simulink model "EPT"  (R2019b)
settings: Solver=FixedStepDiscrete  StartTime=0.0  StopTime=5  FixedStep=0.005  RelTol=1e-3  EnableMultiTasking=on
PreLoadFcn:
  | try, model_open; catch, disp('Error occurred while executing model pre-load callback: model_open.m'); disp('Please assure that the MATLAB working directory is set to the model directory before opening.'); end
InitFcn:
  | try, model_open; catch, end
undefined symbols (not defined in the file or in its folder): Bridge, GCM, H, ln, raptor_get_param_eval, raptor_get_safe_string, raptor_xcp_function
libraries: Raptor_lib x2810, simulink x374, hdlsllib x19
(part 27 of 45)

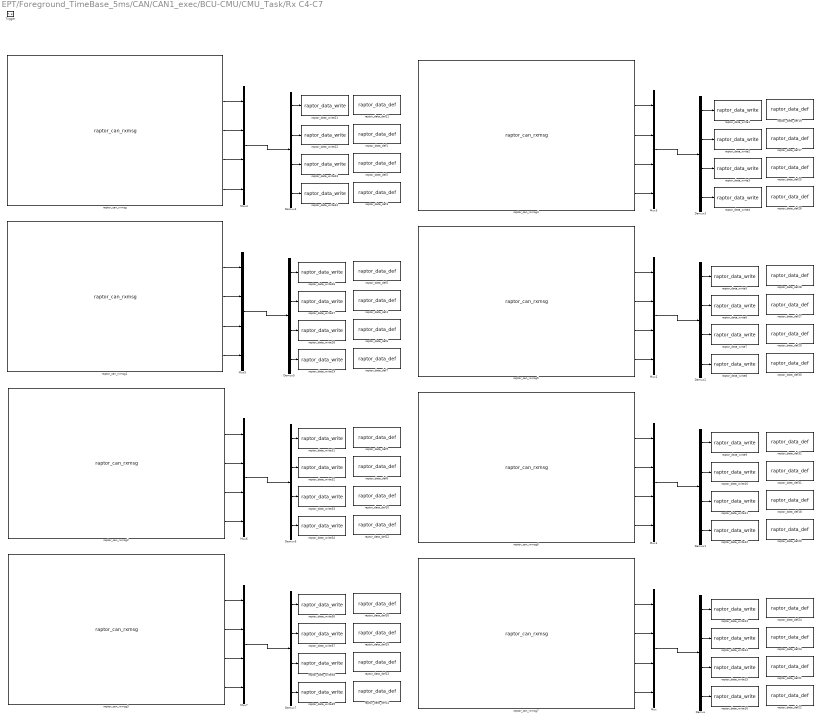
== system EPT/Foreground_TimeBase_5ms/CAN/CAN1_exec/BCU-CMU/CMU_Task/Rx C4-C7 ==
  Trigger : TriggerPort  VariantControl=Variant  PortDimensions=1
  Demux{,1..7} (8 alike) : Demux
  Mux{,1..7} (8 alike) : Mux
  raptor_can_rxmsg : Raptor_lib/CAN/raptor_can_rxmsg  canDefinition=struct('dbcFile', 'CMU1.dbc','message', 'Cell_Temp1','comment', '','signals', {{'Temp1','Temp2','Temp3','Temp4'}},'enabled', [ 1 1 1 1;],'canBus', '''CAN1''','messageID', [ 33604769;],'idMask', [ 536870911;],'payloadMask', [],'payloadValue', [],'period', [ 0;],'mailbox', '''''','queueSize', [ 1;],'label', [ 0;],'ver', [ 2;],'showID', [ 0;],'showRaw', [ 0;],'fill', [ 0;],'editID', [ 0;],'signalOrder', [ 2;])  canBus='CAN1'  mailbox=''  payloadMask=[]  payloadValue=[]  idMask=hex2dec('1FFFFFFF')  queueSize=1  showID=0  label=0  fill=0  id=33604769  showRaw=0  showAge=1  signalOrder=2  signalInfo={{struct('Name', 'Temp1','Startbit', [ 0;],'SignalSize', [ 16;],'ByteOrder', 'BigEndian','ValueType', 'UNSIGNED','Class', 'uint16','Signed', [ 0;],'Factor', [ 0.1;],'Offset', [ -40;],'Min', [ 0;],'Max', [ 0;],'Units', '','Comment', '','StartBit', [ 8;]),struct('Name', 'Temp2','Startbit', [ 0;],'SignalSize', [ 16;],'ByteOrder', 'BigEndian','ValueType', 'UNSIGNED','Class', 'uint16','Signed', [ 0;],'Factor', [ 0.1;],'Offset', [ -40;],'Min', [ 0;],'Max', [ 0;],'Units', '','Comment', '','StartBit', [ 24;]),struct('Name', 'Temp3','Startbit', [ 0;],'SignalSize', [ 16;],'ByteOrder', 'BigEndian','ValueType', 'UNSIGNED','Class', 'uint16','Signed', [ 0;],'Factor', [ 0.1;],'Offset', [ -40;],'Min', [ 0;],'Max', [ 0;],'Units', '','Comment', '','StartBit', [ 40;]),struct('Name', 'Temp4','Startbit', [ 0;],'SignalSize', [ 16;],'ByteOrder', 'BigEndian','ValueType', 'UNSIGNED','Class', 'uint16','Signed', [ 0;],'Factor', [ 0.1;],'Offset', [ -40;],'Min', [ 0;],'Max', [ 0;],'Units', '','Comment', '','StartBit', [ 56;])}}
      settings: SourceProductName=Raptor
  raptor_can_rxmsg1 : Raptor_lib/CAN/raptor_can_rxmsg  canDefinition=struct('dbcFile', 'CMU1.dbc','message', 'Cell_Temp2','comment', '','signals', {{'Temp5','Temp6','Temp7','Temp8'}},'enabled', [ 1 1 1 1;],'canBus', '''CAN1''','messageID', [ 33605025;],'idMask', [ 536870911;],'payloadMask', [],'payloadValue', [],'period', [ 0;],'mailbox', '''''','queueSize', [ 1;],'label', [ 0;],'ver', [ 2;],'showID', [ 0;],'showRaw', [ 0;],'fill', [ 0;],'editID', [ 0;],'signalOrder', [ 2;])  canBus='CAN1'  mailbox=''  payloadMask=[]  payloadValue=[]  idMask=hex2dec('1FFFFFFF')  queueSize=1  showID=0  label=0  fill=0  id=33605025  showRaw=0  showAge=1  signalOrder=2  signalInfo={{struct('Name', 'Temp5','Startbit', [ 0;],'SignalSize', [ 16;],'ByteOrder', 'BigEndian','ValueType', 'UNSIGNED','Class', 'uint16','Signed', [ 0;],'Factor', [ 0.1;],'Offset', [ -40;],'Min', [ 0;],'Max', [ 0;],'Units', '','Comment', '','StartBit', [ 8;]),struct('Name', 'Temp6','Startbit', [ 0;],'SignalSize', [ 16;],'ByteOrder', 'BigEndian','ValueType', 'UNSIGNED','Class', 'uint16','Signed', [ 0;],'Factor', [ 0.1;],'Offset', [ -40;],'Min', [ 0;],'Max', [ 0;],'Units', '','Comment', '','StartBit', [ 24;]),struct('Name', 'Temp7','Startbit', [ 0;],'SignalSize', [ 16;],'ByteOrder', 'BigEndian','ValueType', 'UNSIGNED','Class', 'uint16','Signed', [ 0;],'Factor', [ 0.1;],'Offset', [ -40;],'Min', [ 0;],'Max', [ 0;],'Units', '','Comment', '','StartBit', [ 40;]),struct('Name', 'Temp8','Startbit', [ 0;],'SignalSize', [ 16;],'ByteOrder', 'BigEndian','ValueType', 'UNSIGNED','Class', 'uint16','Signed', [ 0;],'Factor', [ 0.1;],'Offset', [ -40;],'Min', [ 0;],'Max', [ 0;],'Units', '','Comment', '','StartBit', [ 56;])}}
      settings: SourceProductName=Raptor
  raptor_can_rxmsg2 : Raptor_lib/CAN/raptor_can_rxmsg  canDefinition=struct('dbcFile', 'CMU1.dbc','message', 'Cell_Temp3','comment', '','signals', {{'Temp9','Temp10','Temp11','Temp12'}},'enabled', [ 1 1 1 1;],'canBus', '''CAN1''','messageID', [ 33605281;],'idMask', [ 536870911;],'payloadMask', [],'payloadValue', [],'period', [ 0;],'mailbox', '''''','queueSize', [ 1;],'label', [ 0;],'ver', [ 2;],'showID', [ 0;],'showRaw', [ 0;],'fill', [ 0;],'editID', [ 0;],'signalOrder', [ 2;])  canBus='CAN1'  mailbox=''  payloadMask=[]  payloadValue=[]  idMask=hex2dec('1FFFFFFF')  queueSize=1  showID=0  label=0  fill=0  id=33605281  showRaw=0  showAge=1  signalOrder=2  signalInfo={{struct('Name', 'Temp9','Startbit', [ 0;],'SignalSize', [ 16;],'ByteOrder', 'BigEndian','ValueType', 'UNSIGNED','Class', 'uint16','Signed', [ 0;],'Factor', [ 0.1;],'Offset', [ -40;],'Min', [ 0;],'Max', [ 0;],'Units', '','Comment', '','StartBit', [ 8;]),struct('Name', 'Temp10','Startbit', [ 0;],'SignalSize', [ 16;],'ByteOrder', 'BigEndian','ValueType', 'UNSIGNED','Class', 'uint16','Signed', [ 0;],'Factor', [ 0.1;],'Offset', [ -40;],'Min', [ 0;],'Max', [ 0;],'Units', '','Comment', '','StartBit', [ 24;]),struct('Name', 'Temp11','Startbit', [ 0;],'SignalSize', [ 16;],'ByteOrder', 'BigEndian','ValueType', 'UNSIGNED','Class', 'uint16','Signed', [ 0;],'Factor', [ 0.1;],'Offset', [ -40;],'Min', [ 0;],'Max', [ 0;],'Units', '','Comment', '','StartBit', [ 40;]),struct('Name', 'Temp12','Startbit', [ 0;],'SignalSize', [ 16;],'ByteOrder', 'BigEndian','ValueType', 'UNSIGNED','Class', 'uint16','Signed', [ 0;],'Factor', [ 0.1;],'Offset', [ -40;],'Min', [ 0;],'Max', [ 0;],'Units', '','Comment', '','StartBit', [ 56;])}}
      settings: SourceProductName=Raptor
  raptor_can_rxmsg3 : Raptor_lib/CAN/raptor_can_rxmsg  canDefinition=struct('dbcFile', 'CMU1.dbc','message', 'Cell_Temp4','comment', '','signals', {{'Temp13','Temp14','Temp15','Temp16'}},'enabled', [ 1 1 1 1;],'canBus', '''CAN1''','messageID', [ 33605537;],'idMask', [ 536870911;],'payloadMask', [],'payloadValue', [],'period', [ 0;],'mailbox', '''''','queueSize', [ 1;],'label', [ 0;],'ver', [ 2;],'showID', [ 0;],'showRaw', [ 0;],'fill', [ 0;],'editID', [ 0;],'signalOrder', [ 1;])  canBus='CAN1'  mailbox=''  payloadMask=[]  payloadValue=[]  idMask=hex2dec('1FFFFFFF')  queueSize=1  showID=0  label=0  fill=0  id=33605537  showRaw=0  showAge=1  signalOrder=1  signalInfo={{struct('Name', 'Temp13','Startbit', [ 0;],'SignalSize', [ 16;],'ByteOrder', 'BigEndian','ValueType', 'UNSIGNED','Class', 'uint16','Signed', [ 0;],'Factor', [ 0.1;],'Offset', [ -40;],'Min', [ 0;],'Max', [ 0;],'Units', '','Comment', '','StartBit', [ 8;]),struct('Name', 'Temp14','Startbit', [ 0;],'SignalSize', [ 16;],'ByteOrder', 'BigEndian','ValueType', 'UNSIGNED','Class', 'uint16','Signed', [ 0;],'Factor', [ 0.1;],'Offset', [ -40;],'Min', [ 0;],'Max', [ 0;],'Units', '','Comment', '','StartBit', [ 24;]),struct('Name', 'Temp15','Startbit', [ 0;],'SignalSize', [ 16;],'ByteOrder', 'BigEndian','ValueType', 'UNSIGNED','Class', 'uint16','Signed', [ 0;],'Factor', [ 0.1;],'Offset', [ -40;],'Min', [ 0;],'Max', [ 0;],'Units', '','Comment', '','StartBit', [ 40;]),struct('Name', 'Temp16','Startbit', [ 0;],'SignalSize', [ 16;],'ByteOrder', 'BigEndian','ValueType', 'UNSIGNED','Class', 'uint16','Signed', [ 0;],'Factor', [ 0.1;],'Offset', [ -40;],'Min', [ 0;],'Max', [ 0;],'Units', '','Comment', '','StartBit', [ 56;])}}
      settings: SourceProductName=Raptor
  raptor_can_rxmsg4 : Raptor_lib/CAN/raptor_can_rxmsg  canDefinition=struct('dbcFile', 'CMU2.dbc','message', 'Cell_Temp1','comment', '','signals', {{'Temp1','Temp2','Temp3','Temp4'}},'enabled', [ 1 1 1 1;],'canBus', '''CAN1''','messageID', [ 33604770;],'idMask', [ 536870911;],'payloadMask', [],'payloadValue', [],'period', [ 0;],'mailbox', '''''','queueSize', [ 1;],'label', [ 0;],'ver', [ 2;],'showID', [ 0;],'showRaw', [ 0;],'fill', [ 0;],'editID', [ 0;],'signalOrder', [ 2;])  canBus='CAN1'  mailbox=''  payloadMask=[]  payloadValue=[]  idMask=hex2dec('1FFFFFFF')  queueSize=1  showID=0  label=0  fill=0  id=33604770  showRaw=0  showAge=1  signalOrder=2  signalInfo={{struct('Name', 'Temp1','Startbit', [ 0;],'SignalSize', [ 16;],'ByteOrder', 'BigEndian','ValueType', 'UNSIGNED','Class', 'uint16','Signed', [ 0;],'Factor', [ 0.1;],'Offset', [ -40;],'Min', [ 0;],'Max', [ 0;],'Units', '','Comment', '','StartBit', [ 8;]),struct('Name', 'Temp2','Startbit', [ 0;],'SignalSize', [ 16;],'ByteOrder', 'BigEndian','ValueType', 'UNSIGNED','Class', 'uint16','Signed', [ 0;],'Factor', [ 0.1;],'Offset', [ -40;],'Min', [ 0;],'Max', [ 0;],'Units', '','Comment', '','StartBit', [ 24;]),struct('Name', 'Temp3','Startbit', [ 0;],'SignalSize', [ 16;],'ByteOrder', 'BigEndian','ValueType', 'UNSIGNED','Class', 'uint16','Signed', [ 0;],'Factor', [ 0.1;],'Offset', [ -40;],'Min', [ 0;],'Max', [ 0;],'Units', '','Comment', '','StartBit', [ 40;]),struct('Name', 'Temp4','Startbit', [ 0;],'SignalSize', [ 16;],'ByteOrder', 'BigEndian','ValueType', 'UNSIGNED','Class', 'uint16','Signed', [ 0;],'Factor', [ 0.1;],'Offset', [ -40;],'Min', [ 0;],'Max', [ 0;],'Units', '','Comment', '','StartBit', [ 56;])}}
      settings: SourceProductName=Raptor
  raptor_can_rxmsg5 : Raptor_lib/CAN/raptor_can_rxmsg  canDefinition=struct('dbcFile', 'CMU2.dbc','message', 'Cell_Temp2','comment', '','signals', {{'Temp5','Temp6','Temp7','Temp8'}},'enabled', [ 1 1 1 1;],'canBus', '''CAN1''','messageID', [ 33605026;],'idMask', [ 536870911;],'payloadMask', [],'payloadValue', [],'period', [ 0;],'mailbox', '''''','queueSize', [ 1;],'label', [ 0;],'ver', [ 2;],'showID', [ 0;],'showRaw', [ 0;],'fill', [ 0;],'editID', [ 0;],'signalOrder', [ 2;])  canBus='CAN1'  mailbox=''  payloadMask=[]  payloadValue=[]  idMask=hex2dec('1FFFFFFF')  queueSize=1  showID=0  label=0  fill=0  id=33605026  showRaw=0  showAge=1  signalOrder=2  signalInfo={{struct('Name', 'Temp5','Startbit', [ 0;],'SignalSize', [ 16;],'ByteOrder', 'BigEndian','ValueType', 'UNSIGNED','Class', 'uint16','Signed', [ 0;],'Factor', [ 0.1;],'Offset', [ -40;],'Min', [ 0;],'Max', [ 0;],'Units', '','Comment', '','StartBit', [ 8;]),struct('Name', 'Temp6','Startbit', [ 0;],'SignalSize', [ 16;],'ByteOrder', 'BigEndian','ValueType', 'UNSIGNED','Class', 'uint16','Signed', [ 0;],'Factor', [ 0.1;],'Offset', [ -40;],'Min', [ 0;],'Max', [ 0;],'Units', '','Comment', '','StartBit', [ 24;]),struct('Name', 'Temp7','Startbit', [ 0;],'SignalSize', [ 16;],'ByteOrder', 'BigEndian','ValueType', 'UNSIGNED','Class', 'uint16','Signed', [ 0;],'Factor', [ 0.1;],'Offset', [ -40;],'Min', [ 0;],'Max', [ 0;],'Units', '','Comment', '','StartBit', [ 40;]),struct('Name', 'Temp8','Startbit', [ 0;],'SignalSize', [ 16;],'ByteOrder', 'BigEndian','ValueType', 'UNSIGNED','Class', 'uint16','Signed', [ 0;],'Factor', [ 0.1;],'Offset', [ -40;],'Min', [ 0;],'Max', [ 0;],'Units', '','Comment', '','StartBit', [ 56;])}}
      settings: SourceProductName=Raptor
  raptor_can_rxmsg6 : Raptor_lib/CAN/raptor_can_rxmsg  canDefinition=struct('dbcFile', 'CMU2.dbc','message', 'Cell_Temp3','comment', '','signals', {{'Temp9','Temp10','Temp11','Temp12'}},'enabled', [ 1 1 1 1;],'canBus', '''CAN1''','messageID', [ 33605282;],'idMask', [ 536870911;],'payloadMask', [],'payloadValue', [],'period', [ 0;],'mailbox', '''''','queueSize', [ 1;],'label', [ 0;],'ver', [ 2;],'showID', [ 0;],'showRaw', [ 0;],'fill', [ 0;],'editID', [ 0;],'signalOrder', [ 2;])  canBus='CAN1'  mailbox=''  payloadMask=[]  payloadValue=[]  idMask=hex2dec('1FFFFFFF')  queueSize=1  showID=0  label=0  fill=0  id=33605282  showRaw=0  showAge=1  signalOrder=2  signalInfo={{struct('Name', 'Temp9','Startbit', [ 0;],'SignalSize', [ 16;],'ByteOrder', 'BigEndian','ValueType', 'UNSIGNED','Class', 'uint16','Signed', [ 0;],'Factor', [ 0.1;],'Offset', [ -40;],'Min', [ 0;],'Max', [ 0;],'Units', '','Comment', '','StartBit', [ 8;]),struct('Name', 'Temp10','Startbit', [ 0;],'SignalSize', [ 16;],'ByteOrder', 'BigEndian','ValueType', 'UNSIGNED','Class', 'uint16','Signed', [ 0;],'Factor', [ 0.1;],'Offset', [ -40;],'Min', [ 0;],'Max', [ 0;],'Units', '','Comment', '','StartBit', [ 24;]),struct('Name', 'Temp11','Startbit', [ 0;],'SignalSize', [ 16;],'ByteOrder', 'BigEndian','ValueType', 'UNSIGNED','Class', 'uint16','Signed', [ 0;],'Factor', [ 0.1;],'Offset', [ -40;],'Min', [ 0;],'Max', [ 0;],'Units', '','Comment', '','StartBit', [ 40;]),struct('Name', 'Temp12','Startbit', [ 0;],'SignalSize', [ 16;],'ByteOrder', 'BigEndian','ValueType', 'UNSIGNED','Class', 'uint16','Signed', [ 0;],'Factor', [ 0.1;],'Offset', [ -40;],'Min', [ 0;],'Max', [ 0;],'Units', '','Comment', '','StartBit', [ 56;])}}
      settings: SourceProductName=Raptor
  raptor_can_rxmsg7 : Raptor_lib/CAN/raptor_can_rxmsg  canDefinition=struct('dbcFile', 'CMU2.dbc','message', 'Cell_Temp4','comment', '','signals', {{'Temp13','Temp14','Temp15','Temp16'}},'enabled', [ 1 1 1 1;],'canBus', '''CAN1''','messageID', [ 33605538;],'idMask', [ 536870911;],'payloadMask', [],'payloadValue', [],'period', [ 0;],'mailbox', '''''','queueSize', [ 1;],'label', [ 0;],'ver', [ 2;],'showID', [ 0;],'showRaw', [ 0;],'fill', [ 0;],'editID', [ 0;],'signalOrder', [ 2;])  canBus='CAN1'  mailbox=''  payloadMask=[]  payloadValue=[]  idMask=hex2dec('1FFFFFFF')  queueSize=1  showID=0  label=0  fill=0  id=33605538  showRaw=0  showAge=1  signalOrder=2  signalInfo={{struct('Name', 'Temp13','Startbit', [ 0;],'SignalSize', [ 16;],'ByteOrder', 'BigEndian','ValueType', 'UNSIGNED','Class', 'uint16','Signed', [ 0;],'Factor', [ 0.1;],'Offset', [ -40;],'Min', [ 0;],'Max', [ 0;],'Units', '','Comment', '','StartBit', [ 8;]),struct('Name', 'Temp14','Startbit', [ 0;],'SignalSize', [ 16;],'ByteOrder', 'BigEndian','ValueType', 'UNSIGNED','Class', 'uint16','Signed', [ 0;],'Factor', [ 0.1;],'Offset', [ -40;],'Min', [ 0;],'Max', [ 0;],'Units', '','Comment', '','StartBit', [ 24;]),struct('Name', 'Temp15','Startbit', [ 0;],'SignalSize', [ 16;],'ByteOrder', 'BigEndian','ValueType', 'UNSIGNED','Class', 'uint16','Signed', [ 0;],'Factor', [ 0.1;],'Offset', [ -40;],'Min', [ 0;],'Max', [ 0;],'Units', '','Comment', '','StartBit', [ 40;]),struct('Name', 'Temp16','Startbit', [ 0;],'SignalSize', [ 16;],'ByteOrder', 'BigEndian','ValueType', 'UNSIGNED','Class', 'uint16','Signed', [ 0;],'Factor', [ 0.1;],'Offset', [ -40;],'Min', [ 0;],'Max', [ 0;],'Units', '','Comment', '','StartBit', [ 56;])}}
      settings: SourceProductName=Raptor
  raptor_data_def1 : Raptor_lib/Data Storage/raptor_data_def  dataName='CMU1_CELL02_TEMP'  initValue=0  dataType=double  storage=Volatile (RAM)  calVisible=on  calType=Adjustment  calDispType=Number  calEnum={'False', 'True'}  calGain=1.0  calOffset=0  calMin=-inf  calMax=inf  calFormat='2.3'  calUnit=''  calHelp=''  calAccess=1  calFunction=raptor_xcp_function(gcb)  calDispHeaders=off  calColHeaders={'Col1' 'Col2' 'Col3'}  calRowHeaders={'Row1' 'Row2' 'Row3'}
      settings: SourceProductName=Raptor
  raptor_data_def10 : Raptor_lib/Data Storage/raptor_data_def  dataName='CMU1_CELL11_TEMP'  initValue=0  dataType=double  storage=Volatile (RAM)  calVisible=on  calType=Adjustment  calDispType=Number  calEnum={'False', 'True'}  calGain=1.0  calOffset=0  calMin=-inf  calMax=inf  calFormat='2.3'  calUnit=''  calHelp=''  calAccess=1  calFunction=raptor_xcp_function(gcb)  calDispHeaders=off  calColHeaders={'Col1' 'Col2' 'Col3'}  calRowHeaders={'Row1' 'Row2' 'Row3'}
      settings: SourceProductName=Raptor
  raptor_data_def11 : Raptor_lib/Data Storage/raptor_data_def  dataName='CMU1_CELL01_TEMP'  initValue=0  dataType=double  storage=Volatile (RAM)  calVisible=on  calType=Adjustment  calDispType=Number  calEnum={'False', 'True'}  calGain=1.0  calOffset=0  calMin=-inf  calMax=inf  calFormat='2.3'  calUnit=''  calHelp=''  calAccess=1  calFunction=raptor_xcp_function(gcb)  calDispHeaders=off  calColHeaders={'Col1' 'Col2' 'Col3'}  calRowHeaders={'Row1' 'Row2' 'Row3'}
      settings: SourceProductName=Raptor
  raptor_data_def12 : Raptor_lib/Data Storage/raptor_data_def  dataName='CMU1_CELL12_TEMP'  initValue=0  dataType=double  storage=Volatile (RAM)  calVisible=on  calType=Adjustment  calDispType=Number  calEnum={'False', 'True'}  calGain=1.0  calOffset=0  calMin=-inf  calMax=inf  calFormat='2.3'  calUnit=''  calHelp=''  calAccess=1  calFunction=raptor_xcp_function(gcb)  calDispHeaders=off  calColHeaders={'Col1' 'Col2' 'Col3'}  calRowHeaders={'Row1' 'Row2' 'Row3'}
      settings: SourceProductName=Raptor
  raptor_data_def13 : Raptor_lib/Data Storage/raptor_data_def  dataName='CMU1_CELL15_TEMP'  initValue=0  dataType=double  storage=Volatile (RAM)  calVisible=on  calType=Adjustment  calDispType=Number  calEnum={'False', 'True'}  calGain=1.0  calOffset=0  calMin=-inf  calMax=inf  calFormat='2.3'  calUnit=''  calHelp=''  calAccess=1  calFunction=raptor_xcp_function(gcb)  calDispHeaders=off  calColHeaders={'Col1' 'Col2' 'Col3'}  calRowHeaders={'Row1' 'Row2' 'Row3'}
      settings: SourceProductName=Raptor
  raptor_data_def14 : Raptor_lib/Data Storage/raptor_data_def  dataName='CMU1_CELL16_TEMP'  initValue=0  dataType=double  storage=Volatile (RAM)  calVisible=on  calType=Adjustment  calDispType=Number  calEnum={'False', 'True'}  calGain=1.0  calOffset=0  calMin=-inf  calMax=inf  calFormat='2.3'  calUnit=''  calHelp=''  calAccess=1  calFunction=raptor_xcp_function(gcb)  calDispHeaders=off  calColHeaders={'Col1' 'Col2' 'Col3'}  calRowHeaders={'Row1' 'Row2' 'Row3'}
      settings: SourceProductName=Raptor
  raptor_data_def15 : Raptor_lib/Data Storage/raptor_data_def  dataName='CMU1_CELL14_TEMP'  initValue=0  dataType=double  storage=Volatile (RAM)  calVisible=on  calType=Adjustment  calDispType=Number  calEnum={'False', 'True'}  calGain=1.0  calOffset=0  calMin=-inf  calMax=inf  calFormat='2.3'  calUnit=''  calHelp=''  calAccess=1  calFunction=raptor_xcp_function(gcb)  calDispHeaders=off  calColHeaders={'Col1' 'Col2' 'Col3'}  calRowHeaders={'Row1' 'Row2' 'Row3'}
      settings: SourceProductName=Raptor
  raptor_data_def16 : Raptor_lib/Data Storage/raptor_data_def  dataName='CMU1_CELL13_TEMP'  initValue=0  dataType=double  storage=Volatile (RAM)  calVisible=on  calType=Adjustment  calDispType=Number  calEnum={'False', 'True'}  calGain=1.0  calOffset=0  calMin=-inf  calMax=inf  calFormat='2.3'  calUnit=''  calHelp=''  calAccess=1  calFunction=raptor_xcp_function(gcb)  calDispHeaders=off  calColHeaders={'Col1' 'Col2' 'Col3'}  calRowHeaders={'Row1' 'Row2' 'Row3'}
      settings: SourceProductName=Raptor
  raptor_data_def17 : Raptor_lib/Data Storage/raptor_data_def  dataName='CMU2_CELL02_TEMP'  initValue=0  dataType=double  storage=Volatile (RAM)  calVisible=on  calType=Adjustment  calDispType=Number  calEnum={'False', 'True'}  calGain=1.0  calOffset=0  calMin=-inf  calMax=inf  calFormat='2.3'  calUnit=''  calHelp=''  calAccess=1  calFunction=raptor_xcp_function(gcb)  calDispHeaders=off  calColHeaders={'Col1' 'Col2' 'Col3'}  calRowHeaders={'Row1' 'Row2' 'Row3'}
      settings: SourceProductName=Raptor
  raptor_data_def18 : Raptor_lib/Data Storage/raptor_data_def  dataName='CMU2_CELL11_TEMP'  initValue=0  dataType=double  storage=Volatile (RAM)  calVisible=on  calType=Adjustment  calDispType=Number  calEnum={'False', 'True'}  calGain=1.0  calOffset=0  calMin=-inf  calMax=inf  calFormat='2.3'  calUnit=''  calHelp=''  calAccess=1  calFunction=raptor_xcp_function(gcb)  calDispHeaders=off  calColHeaders={'Col1' 'Col2' 'Col3'}  calRowHeaders={'Row1' 'Row2' 'Row3'}
      settings: SourceProductName=Raptor
  raptor_data_def19 : Raptor_lib/Data Storage/raptor_data_def  dataName='CMU2_CELL01_TEMP'  initValue=0  dataType=double  storage=Volatile (RAM)  calVisible=on  calType=Adjustment  calDispType=Number  calEnum={'False', 'True'}  calGain=1.0  calOffset=0  calMin=-inf  calMax=inf  calFormat='2.3'  calUnit=''  calHelp=''  calAccess=1  calFunction=raptor_xcp_function(gcb)  calDispHeaders=off  calColHeaders={'Col1' 'Col2' 'Col3'}  calRowHeaders={'Row1' 'Row2' 'Row3'}
      settings: SourceProductName=Raptor
  raptor_data_def2 : Raptor_lib/Data Storage/raptor_data_def  dataName='CMU1_CELL03_TEMP'  initValue=0  dataType=double  storage=Volatile (RAM)  calVisible=on  calType=Adjustment  calDispType=Number  calEnum={'False', 'True'}  calGain=1.0  calOffset=0  calMin=-inf  calMax=inf  calFormat='2.3'  calUnit=''  calHelp=''  calAccess=1  calFunction=raptor_xcp_function(gcb)  calDispHeaders=off  calColHeaders={'Col1' 'Col2' 'Col3'}  calRowHeaders={'Row1' 'Row2' 'Row3'}
      settings: SourceProductName=Raptor
  raptor_data_def20 : Raptor_lib/Data Storage/raptor_data_def  dataName='CMU2_CELL12_TEMP'  initValue=0  dataType=double  storage=Volatile (RAM)  calVisible=on  calType=Adjustment  calDispType=Number  calEnum={'False', 'True'}  calGain=1.0  calOffset=0  calMin=-inf  calMax=inf  calFormat='2.3'  calUnit=''  calHelp=''  calAccess=1  calFunction=raptor_xcp_function(gcb)  calDispHeaders=off  calColHeaders={'Col1' 'Col2' 'Col3'}  calRowHeaders={'Row1' 'Row2' 'Row3'}
      settings: SourceProductName=Raptor
  raptor_data_def21 : Raptor_lib/Data Storage/raptor_data_def  dataName='CMU2_CELL15_TEMP'  initValue=0  dataType=double  storage=Volatile (RAM)  calVisible=on  calType=Adjustment  calDispType=Number  calEnum={'False', 'True'}  calGain=1.0  calOffset=0  calMin=-inf  calMax=inf  calFormat='2.3'  calUnit=''  calHelp=''  calAccess=1  calFunction=raptor_xcp_function(gcb)  calDispHeaders=off  calColHeaders={'Col1' 'Col2' 'Col3'}  calRowHeaders={'Row1' 'Row2' 'Row3'}
      settings: SourceProductName=Raptor
  raptor_data_def22 : Raptor_lib/Data Storage/raptor_data_def  dataName='CMU2_CELL16_TEMP'  initValue=0  dataType=double  storage=Volatile (RAM)  calVisible=on  calType=Adjustment  calDispType=Number  calEnum={'False', 'True'}  calGain=1.0  calOffset=0  calMin=-inf  calMax=inf  calFormat='2.3'  calUnit=''  calHelp=''  calAccess=1  calFunction=raptor_xcp_function(gcb)  calDispHeaders=off  calColHeaders={'Col1' 'Col2' 'Col3'}  calRowHeaders={'Row1' 'Row2' 'Row3'}
      settings: SourceProductName=Raptor
  raptor_data_def23 : Raptor_lib/Data Storage/raptor_data_def  dataName='CMU2_CELL14_TEMP'  initValue=0  dataType=double  storage=Volatile (RAM)  calVisible=on  calType=Adjustment  calDispType=Number  calEnum={'False', 'True'}  calGain=1.0  calOffset=0  calMin=-inf  calMax=inf  calFormat='2.3'  calUnit=''  calHelp=''  calAccess=1  calFunction=raptor_xcp_function(gcb)  calDispHeaders=off  calColHeaders={'Col1' 'Col2' 'Col3'}  calRowHeaders={'Row1' 'Row2' 'Row3'}
      settings: SourceProductName=Raptor
  raptor_data_def24 : Raptor_lib/Data Storage/raptor_data_def  dataName='CMU2_CELL13_TEMP'  initValue=0  dataType=double  storage=Volatile (RAM)  calVisible=on  calType=Adjustment  calDispType=Number  calEnum={'False', 'True'}  calGain=1.0  calOffset=0  calMin=-inf  calMax=inf  calFormat='2.3'  calUnit=''  calHelp=''  calAccess=1  calFunction=raptor_xcp_function(gcb)  calDispHeaders=off  calColHeaders={'Col1' 'Col2' 'Col3'}  calRowHeaders={'Row1' 'Row2' 'Row3'}
      settings: SourceProductName=Raptor
  raptor_data_def25 : Raptor_lib/Data Storage/raptor_data_def  dataName='CMU2_CELL03_TEMP'  initValue=0  dataType=double  storage=Volatile (RAM)  calVisible=on  calType=Adjustment  calDispType=Number  calEnum={'False', 'True'}  calGain=1.0  calOffset=0  calMin=-inf  calMax=inf  calFormat='2.3'  calUnit=''  calHelp=''  calAccess=1  calFunction=raptor_xcp_function(gcb)  calDispHeaders=off  calColHeaders={'Col1' 'Col2' 'Col3'}  calRowHeaders={'Row1' 'Row2' 'Row3'}
      settings: SourceProductName=Raptor
  raptor_data_def26 : Raptor_lib/Data Storage/raptor_data_def  dataName='CMU2_CELL04_TEMP'  initValue=0  dataType=double  storage=Volatile (RAM)  calVisible=on  calType=Adjustment  calDispType=Number  calEnum={'False', 'True'}  calGain=1.0  calOffset=0  calMin=-inf  calMax=inf  calFormat='2.3'  calUnit=''  calHelp=''  calAccess=1  calFunction=raptor_xcp_function(gcb)  calDispHeaders=off  calColHeaders={'Col1' 'Col2' 'Col3'}  calRowHeaders={'Row1' 'Row2' 'Row3'}
      settings: SourceProductName=Raptor
  raptor_data_def27 : Raptor_lib/Data Storage/raptor_data_def  dataName='CMU2_CELL06_TEMP'  initValue=0  dataType=double  storage=Volatile (RAM)  calVisible=on  calType=Adjustment  calDispType=Number  calEnum={'False', 'True'}  calGain=1.0  calOffset=0  calMin=-inf  calMax=inf  calFormat='2.3'  calUnit=''  calHelp=''  calAccess=1  calFunction=raptor_xcp_function(gcb)  calDispHeaders=off  calColHeaders={'Col1' 'Col2' 'Col3'}  calRowHeaders={'Row1' 'Row2' 'Row3'}
      settings: SourceProductName=Raptor
  raptor_data_def28 : Raptor_lib/Data Storage/raptor_data_def  dataName='CMU2_CELL05_TEMP'  initValue=0  dataType=double  storage=Volatile (RAM)  calVisible=on  calType=Adjustment  calDispType=Number  calEnum={'False', 'True'}  calGain=1.0  calOffset=0  calMin=-inf  calMax=inf  calFormat='2.3'  calUnit=''  calHelp=''  calAccess=1  calFunction=raptor_xcp_function(gcb)  calDispHeaders=off  calColHeaders={'Col1' 'Col2' 'Col3'}  calRowHeaders={'Row1' 'Row2' 'Row3'}
      settings: SourceProductName=Raptor
  raptor_data_def29 : Raptor_lib/Data Storage/raptor_data_def  dataName='CMU2_CELL07_TEMP'  initValue=0  dataType=double  storage=Volatile (RAM)  calVisible=on  calType=Adjustment  calDispType=Number  calEnum={'False', 'True'}  calGain=1.0  calOffset=0  calMin=-inf  calMax=inf  calFormat='2.3'  calUnit=''  calHelp=''  calAccess=1  calFunction=raptor_xcp_function(gcb)  calDispHeaders=off  calColHeaders={'Col1' 'Col2' 'Col3'}  calRowHeaders={'Row1' 'Row2' 'Row3'}
      settings: SourceProductName=Raptor
  raptor_data_def3 : Raptor_lib/Data Storage/raptor_data_def  dataName='CMU1_CELL04_TEMP'  initValue=0  dataType=double  storage=Volatile (RAM)  calVisible=on  calType=Adjustment  calDispType=Number  calEnum={'False', 'True'}  calGain=1.0  calOffset=0  calMin=-inf  calMax=inf  calFormat='2.3'  calUnit=''  calHelp=''  calAccess=1  calFunction=raptor_xcp_function(gcb)  calDispHeaders=off  calColHeaders={'Col1' 'Col2' 'Col3'}  calRowHeaders={'Row1' 'Row2' 'Row3'}
      settings: SourceProductName=Raptor
  raptor_data_def30 : Raptor_lib/Data Storage/raptor_data_def  dataName='CMU2_CELL08_TEMP'  initValue=0  dataType=double  storage=Volatile (RAM)  calVisible=on  calType=Adjustment  calDispType=Number  calEnum={'False', 'True'}  calGain=1.0  calOffset=0  calMin=-inf  calMax=inf  calFormat='2.3'  calUnit=''  calHelp=''  calAccess=1  calFunction=raptor_xcp_function(gcb)  calDispHeaders=off  calColHeaders={'Col1' 'Col2' 'Col3'}  calRowHeaders={'Row1' 'Row2' 'Row3'}
      settings: SourceProductName=Raptor
  raptor_data_def31 : Raptor_lib/Data Storage/raptor_data_def  dataName='CMU2_CELL10_TEMP'  initValue=0  dataType=double  storage=Volatile (RAM)  calVisible=on  calType=Adjustment  calDispType=Number  calEnum={'False', 'True'}  calGain=1.0  calOffset=0  calMin=-inf  calMax=inf  calFormat='2.3'  calUnit=''  calHelp=''  calAccess=1  calFunction=raptor_xcp_function(gcb)  calDispHeaders=off  calColHeaders={'Col1' 'Col2' 'Col3'}  calRowHeaders={'Row1' 'Row2' 'Row3'}
      settings: SourceProductName=Raptor
  raptor_data_def32 : Raptor_lib/Data Storage/raptor_data_def  dataName='CMU2_CELL09_TEMP'  initValue=0  dataType=double  storage=Volatile (RAM)  calVisible=on  calType=Adjustment  calDispType=Number  calEnum={'False', 'True'}  calGain=1.0  calOffset=0  calMin=-inf  calMax=inf  calFormat='2.3'  calUnit=''  calHelp=''  calAccess=1  calFunction=raptor_xcp_function(gcb)  calDispHeaders=off  calColHeaders={'Col1' 'Col2' 'Col3'}  calRowHeaders={'Row1' 'Row2' 'Row3'}
      settings: SourceProductName=Raptor
  raptor_data_def4 : Raptor_lib/Data Storage/raptor_data_def  dataName='CMU1_CELL06_TEMP'  initValue=0  dataType=double  storage=Volatile (RAM)  calVisible=on  calType=Adjustment  calDispType=Number  calEnum={'False', 'True'}  calGain=1.0  calOffset=0  calMin=-inf  calMax=inf  calFormat='2.3'  calUnit=''  calHelp=''  calAccess=1  calFunction=raptor_xcp_function(gcb)  calDispHeaders=off  calColHeaders={'Col1' 'Col2' 'Col3'}  calRowHeaders={'Row1' 'Row2' 'Row3'}
      settings: SourceProductName=Raptor
  raptor_data_def5 : Raptor_lib/Data Storage/raptor_data_def  dataName='CMU1_CELL05_TEMP'  initValue=0  dataType=double  storage=Volatile (RAM)  calVisible=on  calType=Adjustment  calDispType=Number  calEnum={'False', 'True'}  calGain=1.0  calOffset=0  calMin=-inf  calMax=inf  calFormat='2.3'  calUnit=''  calHelp=''  calAccess=1  calFunction=raptor_xcp_function(gcb)  calDispHeaders=off  calColHeaders={'Col1' 'Col2' 'Col3'}  calRowHeaders={'Row1' 'Row2' 'Row3'}
      settings: SourceProductName=Raptor
  raptor_data_def6 : Raptor_lib/Data Storage/raptor_data_def  dataName='CMU1_CELL07_TEMP'  initValue=0  dataType=double  storage=Volatile (RAM)  calVisible=on  calType=Adjustment  calDispType=Number  calEnum={'False', 'True'}  calGain=1.0  calOffset=0  calMin=-inf  calMax=inf  calFormat='2.3'  calUnit=''  calHelp=''  calAccess=1  calFunction=raptor_xcp_function(gcb)  calDispHeaders=off  calColHeaders={'Col1' 'Col2' 'Col3'}  calRowHeaders={'Row1' 'Row2' 'Row3'}
      settings: SourceProductName=Raptor
  raptor_data_def7 : Raptor_lib/Data Storage/raptor_data_def  dataName='CMU1_CELL08_TEMP'  initValue=0  dataType=double  storage=Volatile (RAM)  calVisible=on  calType=Adjustment  calDispType=Number  calEnum={'False', 'True'}  calGain=1.0  calOffset=0  calMin=-inf  calMax=inf  calFormat='2.3'  calUnit=''  calHelp=''  calAccess=1  calFunction=raptor_xcp_function(gcb)  calDispHeaders=off  calColHeaders={'Col1' 'Col2' 'Col3'}  calRowHeaders={'Row1' 'Row2' 'Row3'}
      settings: SourceProductName=Raptor
  raptor_data_def8 : Raptor_lib/Data Storage/raptor_data_def  dataName='CMU1_CELL10_TEMP'  initValue=0  dataType=double  storage=Volatile (RAM)  calVisible=on  calType=Adjustment  calDispType=Number  calEnum={'False', 'True'}  calGain=1.0  calOffset=0  calMin=-inf  calMax=inf  calFormat='2.3'  calUnit=''  calHelp=''  calAccess=1  calFunction=raptor_xcp_function(gcb)  calDispHeaders=off  calColHeaders={'Col1' 'Col2' 'Col3'}  calRowHeaders={'Row1' 'Row2' 'Row3'}
      settings: SourceProductName=Raptor
  raptor_data_def9 : Raptor_lib/Data Storage/raptor_data_def  dataName='CMU1_CELL09_TEMP'  initValue=0  dataType=double  storage=Volatile (RAM)  calVisible=on  calType=Adjustment  calDispType=Number  calEnum={'False', 'True'}  calGain=1.0  calOffset=0  calMin=-inf  calMax=inf  calFormat='2.3'  calUnit=''  calHelp=''  calAccess=1  calFunction=raptor_xcp_function(gcb)  calDispHeaders=off  calColHeaders={'Col1' 'Col2' 'Col3'}  calRowHeaders={'Row1' 'Row2' 'Row3'}
      settings: SourceProductName=Raptor
  raptor_data_write1 : Raptor_lib/Data Storage/raptor_data_write  dataName='CMU2_CELL01_TEMP'  dataShape=Scalar  idxSource=Input Port  idxRow=1  idxCol=1
      settings: SourceProductName=Raptor
  raptor_data_write10 : Raptor_lib/Data Storage/raptor_data_write  dataName='CMU2_CELL10_TEMP'  dataShape=Scalar  idxSource=Input Port  idxRow=1  idxCol=1
      settings: SourceProductName=Raptor
  raptor_data_write11 : Raptor_lib/Data Storage/raptor_data_write  dataName='CMU2_CELL11_TEMP'  dataShape=Scalar  idxSource=Input Port  idxRow=1  idxCol=1
      settings: SourceProductName=Raptor
  raptor_data_write12 : Raptor_lib/Data Storage/raptor_data_write  dataName='CMU2_CELL12_TEMP'  dataShape=Scalar  idxSource=Input Port  idxRow=1  idxCol=1
      settings: SourceProductName=Raptor
  raptor_data_write13 : Raptor_lib/Data Storage/raptor_data_write  dataName='CMU2_CELL13_TEMP'  dataShape=Scalar  idxSource=Input Port  idxRow=1  idxCol=1
      settings: SourceProductName=Raptor
  raptor_data_write14 : Raptor_lib/Data Storage/raptor_data_write  dataName='CMU2_CELL14_TEMP'  dataShape=Scalar  idxSource=Input Port  idxRow=1  idxCol=1
      settings: SourceProductName=Raptor
  raptor_data_write15 : Raptor_lib/Data Storage/raptor_data_write  dataName='CMU2_CELL15_TEMP'  dataShape=Scalar  idxSource=Input Port  idxRow=1  idxCol=1
      settings: SourceProductName=Raptor
  raptor_data_write16 : Raptor_lib/Data Storage/raptor_data_write  dataName='CMU2_CELL16_TEMP'  dataShape=Scalar  idxSource=Input Port  idxRow=1  idxCol=1
      settings: SourceProductName=Raptor
  raptor_data_write2 : Raptor_lib/Data Storage/raptor_data_write  dataName='CMU2_CELL02_TEMP'  dataShape=Scalar  idxSource=Input Port  idxRow=1  idxCol=1
      settings: SourceProductName=Raptor
  raptor_data_write21 : Raptor_lib/Data Storage/raptor_data_write  dataName='CMU1_CELL01_TEMP'  dataShape=Scalar  idxSource=Input Port  idxRow=1  idxCol=1
      settings: SourceProductName=Raptor
  raptor_data_write22 : Raptor_lib/Data Storage/raptor_data_write  dataName='CMU1_CELL02_TEMP'  dataShape=Scalar  idxSource=Input Port  idxRow=1  idxCol=1
      settings: SourceProductName=Raptor
  raptor_data_write23 : Raptor_lib/Data Storage/raptor_data_write  dataName='CMU1_CELL03_TEMP'  dataShape=Scalar  idxSource=Input Port  idxRow=1  idxCol=1
      settings: SourceProductName=Raptor
  raptor_data_write24 : Raptor_lib/Data Storage/raptor_data_write  dataName='CMU1_CELL04_TEMP'  dataShape=Scalar  idxSource=Input Port  idxRow=1  idxCol=1
      settings: SourceProductName=Raptor
  raptor_data_write26 : Raptor_lib/Data Storage/raptor_data_write  dataName='CMU1_CELL05_TEMP'  dataShape=Scalar  idxSource=Input Port  idxRow=1  idxCol=1
      settings: SourceProductName=Raptor
  raptor_data_write27 : Raptor_lib/Data Storage/raptor_data_write  dataName='CMU1_CELL06_TEMP'  dataShape=Scalar  idxSource=Input Port  idxRow=1  idxCol=1
      settings: SourceProductName=Raptor
  raptor_data_write28 : Raptor_lib/Data Storage/raptor_data_write  dataName='CMU1_CELL07_TEMP'  dataShape=Scalar  idxSource=Input Port  idxRow=1  idxCol=1
      settings: SourceProductName=Raptor
  raptor_data_write29 : Raptor_lib/Data Storage/raptor_data_write  dataName='CMU1_CELL08_TEMP'  dataShape=Scalar  idxSource=Input Port  idxRow=1  idxCol=1
      settings: SourceProductName=Raptor
  raptor_data_write3 : Raptor_lib/Data Storage/raptor_data_write  dataName='CMU2_CELL03_TEMP'  dataShape=Scalar  idxSource=Input Port  idxRow=1  idxCol=1
      settings: SourceProductName=Raptor
  raptor_data_write31 : Raptor_lib/Data Storage/raptor_data_write  dataName='CMU1_CELL09_TEMP'  dataShape=Scalar  idxSource=Input Port  idxRow=1  idxCol=1
      settings: SourceProductName=Raptor
  raptor_data_write32 : Raptor_lib/Data Storage/raptor_data_write  dataName='CMU1_CELL10_TEMP'  dataShape=Scalar  idxSource=Input Port  idxRow=1  idxCol=1
      settings: SourceProductName=Raptor
  raptor_data_write33 : Raptor_lib/Data Storage/raptor_data_write  dataName='CMU1_CELL11_TEMP'  dataShape=Scalar  idxSource=Input Port  idxRow=1  idxCol=1
      settings: SourceProductName=Raptor
  raptor_data_write34 : Raptor_lib/Data Storage/raptor_data_write  dataName='CMU1_CELL12_TEMP'  dataShape=Scalar  idxSource=Input Port  idxRow=1  idxCol=1
      settings: SourceProductName=Raptor
  raptor_data_write36 : Raptor_lib/Data Storage/raptor_data_write  dataName='CMU1_CELL13_TEMP'  dataShape=Scalar  idxSource=Input Port  idxRow=1  idxCol=1
      settings: SourceProductName=Raptor
  raptor_data_write37 : Raptor_lib/Data Storage/raptor_data_write  dataName='CMU1_CELL14_TEMP'  dataShape=Scalar  idxSource=Input Port  idxRow=1  idxCol=1
      settings: SourceProductName=Raptor
  raptor_data_write38 : Raptor_lib/Data Storage/raptor_data_write  dataName='CMU1_CELL15_TEMP'  dataShape=Scalar  idxSource=Input Port  idxRow=1  idxCol=1
      settings: SourceProductName=Raptor
  raptor_data_write39 : Raptor_lib/Data Storage/raptor_data_write  dataName='CMU1_CELL16_TEMP'  dataShape=Scalar  idxSource=Input Port  idxRow=1  idxCol=1
      settings: SourceProductName=Raptor
  raptor_data_write4 : Raptor_lib/Data Storage/raptor_data_write  dataName='CMU2_CELL04_TEMP'  dataShape=Scalar  idxSource=Input Port  idxRow=1  idxCol=1
      settings: SourceProductName=Raptor
  raptor_data_write5 : Raptor_lib/Data Storage/raptor_data_write  dataName='CMU2_CELL05_TEMP'  dataShape=Scalar  idxSource=Input Port  idxRow=1  idxCol=1
      settings: SourceProductName=Raptor
  raptor_data_write6 : Raptor_lib/Data Storage/raptor_data_write  dataName='CMU2_CELL06_TEMP'  dataShape=Scalar  idxSource=Input Port  idxRow=1  idxCol=1
      settings: SourceProductName=Raptor
  raptor_data_write7 : Raptor_lib/Data Storage/raptor_data_write  dataName='CMU2_CELL07_TEMP'  dataShape=Scalar  idxSource=Input Port  idxRow=1  idxCol=1
      settings: SourceProductName=Raptor
  raptor_data_write8 : Raptor_lib/Data Storage/raptor_data_write  dataName='CMU2_CELL08_TEMP'  dataShape=Scalar  idxSource=Input Port  idxRow=1  idxCol=1
      settings: SourceProductName=Raptor
  raptor_data_write9 : Raptor_lib/Data Storage/raptor_data_write  dataName='CMU2_CELL09_TEMP'  dataShape=Scalar  idxSource=Input Port  idxRow=1  idxCol=1
      settings: SourceProductName=Raptor
  wires:
  Demux/2 -> raptor_data_write14/1
  raptor_can_rxmsg7/4 -> Mux/3
  raptor_can_rxmsg7/5 -> Mux/4
  raptor_can_rxmsg7/3 -> Mux/2
  Demux/1 -> raptor_data_write13/1
  Mux/1 -> Demux/1
  Demux/4 -> raptor_data_write16/1
  raptor_can_rxmsg7/2 -> Mux/1
  Demux/3 -> raptor_data_write15/1
  Demux1/3 -> raptor_data_write11/1
  Demux1/4 -> raptor_data_write12/1
  raptor_can_rxmsg6/5 -> Mux1/4
  Demux1/2 -> raptor_data_write10/1
  raptor_can_rxmsg6/4 -> Mux1/3
  Demux1/1 -> raptor_data_write9/1
  raptor_can_rxmsg6/2 -> Mux1/1
  Mux1/1 -> Demux1/1
  raptor_can_rxmsg6/3 -> Mux1/2
  Demux2/3 -> raptor_data_write7/1
  Demux2/4 -> raptor_data_write8/1
  raptor_can_rxmsg5/5 -> Mux2/4
  Demux2/2 -> raptor_data_write6/1
  raptor_can_rxmsg5/4 -> Mux2/3
  Demux2/1 -> raptor_data_write5/1
  raptor_can_rxmsg5/2 -> Mux2/1
  Mux2/1 -> Demux2/1
  raptor_can_rxmsg5/3 -> Mux2/2
  Demux3/3 -> raptor_data_write3/1
  Demux3/4 -> raptor_data_write4/1
  raptor_can_rxmsg4/5 -> Mux3/4
  Demux3/2 -> raptor_data_write2/1
  raptor_can_rxmsg4/4 -> Mux3/3
  Demux3/1 -> raptor_data_write1/1
  raptor_can_rxmsg4/2 -> Mux3/1
  Mux3/1 -> Demux3/1
  raptor_can_rxmsg4/3 -> Mux3/2
  Demux4/3 -> raptor_data_write23/1
  Demux4/4 -> raptor_data_write24/1
  raptor_can_rxmsg/5 -> Mux4/4
  Demux4/2 -> raptor_data_write22/1
  raptor_can_rxmsg/4 -> Mux4/3
  Demux4/1 -> raptor_data_write21/1
  raptor_can_rxmsg/2 -> Mux4/1
  Mux4/1 -> Demux4/1
  raptor_can_rxmsg/3 -> Mux4/2
  Demux5/3 -> raptor_data_write28/1
  Demux5/4 -> raptor_data_write29/1
  raptor_can_rxmsg1/5 -> Mux5/4
  Demux5/2 -> raptor_data_write27/1
  raptor_can_rxmsg1/4 -> Mux5/3
  Demux5/1 -> raptor_data_write26/1
  raptor_can_rxmsg1/2 -> Mux5/1
  Mux5/1 -> Demux5/1
  raptor_can_rxmsg1/3 -> Mux5/2
  Demux6/3 -> raptor_data_write33/1
  Demux6/4 -> raptor_data_write34/1
  raptor_can_rxmsg2/5 -> Mux6/4
  Demux6/2 -> raptor_data_write32/1
  raptor_can_rxmsg2/4 -> Mux6/3
  Demux6/1 -> raptor_data_write31/1
  raptor_can_rxmsg2/2 -> Mux6/1
  Mux6/1 -> Demux6/1
  raptor_can_rxmsg2/3 -> Mux6/2
  Demux7/3 -> raptor_data_write38/1
  Demux7/4 -> raptor_data_write39/1
  raptor_can_rxmsg3/5 -> Mux7/4
  Demux7/2 -> raptor_data_write37/1
  raptor_can_rxmsg3/4 -> Mux7/3
  Demux7/1 -> raptor_data_write36/1
  raptor_can_rxmsg3/2 -> Mux7/1
  Mux7/1 -> Demux7/1
  raptor_can_rxmsg3/3 -> Mux7/2

== system EPT/Foreground_TimeBase_5ms/CAN/CAN1_exec/BCU-CMU/CMU_Task/Tx B0-B1 ==
  Trigger : TriggerPort  VariantControl=Variant  PortDimensions=1
  Constant2 : Constant  Value=2
  Constant3 : Constant  Value=hex2dec('A0')
  Constant4 : Constant  Value=hex2dec('B0')
  raptor_can_txmsg : Raptor_lib/CAN/raptor_can_txmsg  canDefinition=struct('dbcFile', 'CMU_CMD.dbc','message', 'HostReadCMD','comment', '','signals', {{'CMU_ID','Offset','Function_Index','ID','LifeCycle'}},'enabled', [ 1 1 1 1 1;],'canBus', '''CAN1''','messageID', [ 16838272;],'idMask', [ 536870911;],'payloadMask', [],'payloadValue', [],'period', [ 0;],'mailbox', '','queueSize', [ 1;],'label', [ 0;],'ver', [ 2;],'showID', [ 0;],'showRaw', [ 0;],'fill', [ 0;],'editID', [ 0;],'signalOrder', [ 2;])  canBus='CAN1'  queueSize=1  payloadMask=[]  payloadValue=[]  period=0  showID=0  label=0  idMask=hex2dec('1FFFFFFF')  fill=0  id=16838272  showRaw=0  signalOrder=2  signalInfo={{struct('Name', 'CMU_ID','Startbit', [ 0;],'SignalSize', [ 8;],'ByteOrder', 'LittleEndian','ValueType', 'UNSIGNED','Class', 'uint8','Signed', [ 0;],'Factor', [ 1;],'Offset', [ 0;],'Min', [ 0;],'Max', [ 0;],'Units', '','Comment', '','StartBit', [ 0;]),struct('Name', 'Offset','Startbit', [ 0;],'SignalSize', [ 8;],'ByteOrder', 'LittleEndian','ValueType', 'UNSIGNED','Class', 'uint8','Signed', [ 0;],'Factor', [ 1;],'Offset', [ 0;],'Min', [ 0;],'Max', [ 0;],'Units', '','Comment', '','StartBit', [ 32;]),struct('Name', 'Function_Index','Startbit', [ 0;],'SignalSize', [ 8;],'ByteOrder', 'LittleEndian','ValueType', 'UNSIGNED','Class', 'uint8','Signed', [ 0;],'Factor', [ 1;],'Offset', [ 0;],'Min', [ 0;],'Max', [ 0;],'Units', '','Comment', '','StartBit', [ 40;]),struct('Name', 'LifeCycle','Startbit', [ 0;],'SignalSize', [ 4;],'ByteOrder', 'LittleEndian','ValueType', 'UNSIGNED','Class', 'uint8','Signed', [ 0;],'Factor', [ 1;],'Offset', [ 0;],'Min', [ 0;],'Max', [ 0;],'Units', '','Comment', '','StartBit', [ 60;]),struct('Name', 'ID','Startbit', [ 0;],'SignalSize', [ 4;],'ByteOrder', 'LittleEndian','ValueType', 'UNSIGNED','Class', 'uint8','Signed', [ 0;],'Factor', [ 1;],'Offset', [ 0;],'Min', [ 0;],'Max', [ 0;],'Units', '','Comment', '','StartBit', [ 56;])}}
      settings: SourceProductName=Raptor
  raptor_data_read2 : Raptor_lib/Data Storage/raptor_data_read  dataName='EPT_RDCMD_RC'  dataShape=Scalar  idxSource=Input  idxRow=1  idxCol=1
      settings: SourceProductName=Raptor
  raptor_data_read4 : Raptor_lib/Data Storage/raptor_data_read  dataName='EPT_RDCMD_HOST_ID'  dataShape=Scalar  idxSource=Input  idxRow=1  idxCol=1
      settings: SourceProductName=Raptor
  wires:
  raptor_data_read4/1 -> raptor_can_txmsg/4  "ID"
  Constant4/1 -> raptor_can_txmsg/3  "Function_Index"
  raptor_data_read2/1 -> raptor_can_txmsg/5  "LifeCycle"
  Constant3/1 -> raptor_can_txmsg/1  "CMU_ID"
  Constant2/1 -> raptor_can_txmsg/2  "Offset"

== system EPT/Foreground_TimeBase_5ms/CAN/CAN1_exec/BCU-CMU/CMU_Task/Tx B2&(BA-BB) ==
  Trigger : TriggerPort  VariantControl=Variant  PortDimensions=1
  Bitwise Operator : simulink/Logic and Bit Operations/Bitwise Operator  logicop=AND  UseBitMask=on  BitMask=bin2dec('01111110')  BitMaskRealWorld=Stored Integer
  Bitwise Operator1 : simulink/Logic and Bit Operations/Bitwise Operator  logicop=AND  UseBitMask=on  BitMask=bin2dec('01111110')  BitMaskRealWorld=Stored Integer
  Constant : Constant  Value=hex2dec('A0')
  Constant1 : Constant  Value=hex2dec('B2')
  Constant3 : Constant  Value=3
  Constant4 : Constant
  Data Type Conversion{,1..3} (4 alike) : DataTypeConversion  OutDataTypeStr=uint8
  IsPositive : simulink/Logic and Bit Operations/Compare To Zero  relop=>  OutDataTypeStr=boolean
  IsPositive1 : simulink/Logic and Bit Operations/Compare To Zero  relop=>  OutDataTypeStr=boolean
  Logical Operator : Logic  Operator=OR  AllPortsSameDT=off  OutDataTypeStr=boolean
  Switch : Switch  Criteria=u2 > Threshold
  raptor_can_txmsg : Raptor_lib/CAN/raptor_can_txmsg  canDefinition=struct('dbcFile', 'CMU_CMD.dbc','message', 'HostReadCMD','comment', '','signals', {{'CMU_ID','Offset','Function_Index','ID','LifeCycle'}},'enabled', [ 1 1 1 1 1;],'canBus', '''CAN1''','messageID', [ 16838272;],'idMask', [ 536870911;],'payloadMask', [],'payloadValue', [],'period', [ 0;],'mailbox', '','queueSize', [ 1;],'label', [ 1;],'ver', [ 2;],'showID', [ 0;],'showRaw', [ 0;],'fill', [ 0;],'editID', [ 0;],'signalOrder', [ 2;])  canBus='CAN1'  queueSize=1  payloadMask=[]  payloadValue=[]  period=0  showID=0  label=1  idMask=hex2dec('1FFFFFFF')  fill=0  id=16838272  showRaw=0  signalOrder=2  signalInfo={{struct('Name', 'CMU_ID','Startbit', [ 0;],'SignalSize', [ 8;],'ByteOrder', 'LittleEndian','ValueType', 'UNSIGNED','Class', 'uint8','Signed', [ 0;],'Factor', [ 1;],'Offset', [ 0;],'Min', [ 0;],'Max', [ 0;],'Units', '','Comment', '','StartBit', [ 0;]),struct('Name', 'Offset','Startbit', [ 0;],'SignalSize', [ 8;],'ByteOrder', 'LittleEndian','ValueType', 'UNSIGNED','Class', 'uint8','Signed', [ 0;],'Factor', [ 1;],'Offset', [ 0;],'Min', [ 0;],'Max', [ 0;],'Units', '','Comment', '','StartBit', [ 32;]),struct('Name', 'Function_Index','Startbit', [ 0;],'SignalSize', [ 8;],'ByteOrder', 'LittleEndian','ValueType', 'UNSIGNED','Class', 'uint8','Signed', [ 0;],'Factor', [ 1;],'Offset', [ 0;],'Min', [ 0;],'Max', [ 0;],'Units', '','Comment', '','StartBit', [ 40;]),struct('Name', 'LifeCycle','Startbit', [ 0;],'SignalSize', [ 4;],'ByteOrder', 'LittleEndian','ValueType', 'UNSIGNED','Class', 'uint8','Signed', [ 0;],'Factor', [ 1;],'Offset', [ 0;],'Min', [ 0;],'Max', [ 0;],'Units', '','Comment', '','StartBit', [ 60;]),struct('Name', 'ID','Startbit', [ 0;],'SignalSize', [ 4;],'ByteOrder', 'LittleEndian','ValueType', 'UNSIGNED','Class', 'uint8','Signed', [ 0;],'Factor', [ 1;],'Offset', [ 0;],'Min', [ 0;],'Max', [ 0;],'Units', '','Comment', '','StartBit', [ 56;])}}
      settings: SourceProductName=Raptor
  raptor_data_read1 : Raptor_lib/Data Storage/raptor_data_read  dataName='EPT_RDCMD_RC'  dataShape=Scalar  idxSource=Input  idxRow=1  idxCol=1
      settings: SourceProductName=Raptor
  raptor_data_read2 : Raptor_lib/Data Storage/raptor_data_read  dataName='CMU1_STATUS'  dataShape=Scalar  idxSource=Input  idxRow=1  idxCol=1
      settings: SourceProductName=Raptor
  raptor_data_read3 : Raptor_lib/Data Storage/raptor_data_read  dataName='CMU2_STATUS'  dataShape=Scalar  idxSource=Input  idxRow=1  idxCol=1
      settings: SourceProductName=Raptor
  raptor_data_read4 : Raptor_lib/Data Storage/raptor_data_read  dataName='EPT_RDCMD_HOST_ID'  dataShape=Scalar  idxSource=Input  idxRow=1  idxCol=1
      settings: SourceProductName=Raptor
  raptor_data_write2 : Raptor_lib/Data Storage/raptor_data_write  dataName='Fault_CMU'  dataShape=Scalar  idxSource=Input Port  idxRow=1  idxCol=1
      settings: SourceProductName=Raptor
  raptor_override : Raptor_lib/Data Storage/raptor_override  paramName='Cal_Fault_CMU'  nameSource=Parameter  measurement=None  calDispType=Number  calEnum={'False', 'True'}  calGain=1.0  calOffset=0.0  calMax=inf  calMin=-inf  calFormat='-1'  calUnit=''  calHelp=''  calAccess=1  calFunction=[raptor_xcp_function(gcb) '|' raptor_get_param_eval(gcb, 'paramName') '_Override']
      settings: SourceProductName=Raptor
  wires:
  Data Type Conversion1/1 -> Bitwise Operator/1
  Bitwise Operator/1 -> Data Type Conversion/1
  raptor_data_read2/1 -> Data Type Conversion1/1
  Bitwise Operator1/1 -> Data Type Conversion2/1
  Data Type Conversion3/1 -> Bitwise Operator1/1
  raptor_data_read3/1 -> Data Type Conversion3/1
  Data Type Conversion/1 -> IsPositive/1
  Data Type Conversion2/1 -> IsPositive1/1
  IsPositive/1 -> Logical Operator/1
  IsPositive1/1 -> Logical Operator/2
  Constant3/1 -> Switch/1
  Constant4/1 -> Switch/3
  Logical Operator/1 -> raptor_override/1
  raptor_data_read1/1 -> raptor_can_txmsg/5  "LifeCycle"
  Switch/1 -> raptor_can_txmsg/2  "Offset"
  Constant/1 -> raptor_can_txmsg/1  "CMU_ID"
  Constant1/1 -> raptor_can_txmsg/3  "Function_Index"
  raptor_data_read4/1 -> raptor_can_txmsg/4  "ID"
  raptor_override/1 -> raptor_data_write2/1, Switch/2
